simulink subsystem "AnalogInputFiltering"  (R2019b)
settings: Solver=VariableStepAuto  StartTime=0.0  StopTime=10.0  RelTol=1e-3
undefined symbols (not defined in the file): boardTempTemperatureCal_mC, boardTempVoltageCal_mV, motorDriverTempTemperatureCal_mC, motorDriverTempVoltageCal_mV, throttlePos1Max_cnt, throttlePos1Min_cnt, throttlePos2Max_cnt, throttlePos2Min_cnt
libraries: eeGeneralControl x2, Map x2, dspstat3 x2
settings Model: Creator=Nick  LastModifiedBy=Nick

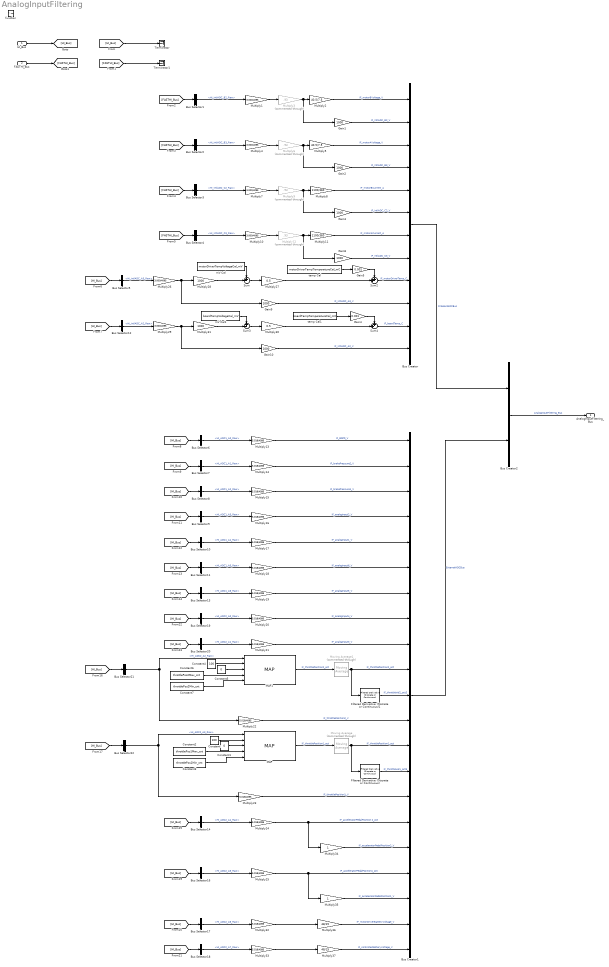
== system AnalogInputFiltering ==
  HI_Bus : Inport
  FASTHI_Bus : Inport  Port=2
  function : TriggerPort  TriggerType=function-call  VariantControl=Variant
  Bus Creator : BusCreator  Inputs=12
  Bus Creator1 : BusCreator  Inputs=21
  Bus Creator2 : BusCreator  Inputs=2
  Bus Selector1 : BusSelector  OutputSignals=HI_intlADC_B2_Raw
  Bus Selector10 : BusSelector  OutputSignals=SPIBus.ADC1Bus.HI_ADC1_A4_Raw
  Bus Selector11 : BusSelector  OutputSignals=SPIBus.ADC1Bus.HI_ADC1_A5_Raw
  Bus Selector12 : BusSelector  OutputSignals=AnalogBus.HI_intlADC_A2_Raw
  Bus Selector13 : BusSelector  OutputSignals=SPIBus.ADC1Bus.HI_ADC1_A6_Raw
  Bus Selector14 : BusSelector  OutputSignals=SPIBus.ADC2Bus.HI_ADC2_A4_Raw
  Bus Selector16 : BusSelector  OutputSignals=SPIBus.ADC2Bus.HI_ADC2_A5_Raw
  Bus Selector17 : BusSelector  OutputSignals=SPIBus.ADC2Bus.HI_ADC2_A6_Raw
  Bus Selector18 : BusSelector  OutputSignals=SPIBus.ADC2Bus.HI_ADC2_A7_Raw
  Bus Selector19 : BusSelector  OutputSignals=SPIBus.ADC2Bus.HI_ADC2_A0_Raw
  Bus Selector2 : BusSelector  OutputSignals=HI_intlADC_B3_Raw
  Bus Selector20 : BusSelector  OutputSignals=SPIBus.ADC2Bus.HI_ADC2_A1_Raw
  Bus Selector21 : BusSelector  OutputSignals=SPIBus.ADC2Bus.HI_ADC2_A2_Raw
  Bus Selector22 : BusSelector  OutputSignals=SPIBus.ADC2Bus.HI_ADC2_A3_Raw
  Bus Selector3 : BusSelector  OutputSignals=HI_intlADC_C2_Raw
  Bus Selector4 : BusSelector  OutputSignals=HI_intlADC_C3_Raw
  Bus Selector5 : BusSelector  OutputSignals=AnalogBus.HI_intlADC_A3_Raw
  Bus Selector6 : BusSelector  OutputSignals=SPIBus.ADC1Bus.HI_ADC1_A0_Raw
  Bus Selector7 : BusSelector  OutputSignals=SPIBus.ADC1Bus.HI_ADC1_A1_Raw
  Bus Selector8 : BusSelector  OutputSignals=SPIBus.ADC1Bus.HI_ADC1_A2_Raw
  Bus Selector9 : BusSelector  OutputSignals=SPIBus.ADC1Bus.HI_ADC1_A3_Raw
  Constant : Constant  Value=100
  Constant1 : Constant  Value=0
  Constant2 : Constant  Value=throttlePos1Max_cnt
  Constant3 : Constant  Value=throttlePos1Min_cnt
  Constant4 : Constant  Value=100
  Constant5 : Constant  Value=0
  Constant6 : Constant  Value=throttlePos2Max_cnt
  Constant7 : Constant  Value=throttlePos2Min_cnt
  Filtered Derivative (Discrete or Continuous) : eeGeneralControl/Filtered Derivative (Discrete or Continuous)  K=1  T=0.01  B=inf  A=-inf  minRatio=10  Ts=-1
      settings: SourceProductName=Simscape Electrical  SourceProductBaseCode=PS
  Filtered Derivative (Discrete or Continuous)1 : eeGeneralControl/Filtered Derivative (Discrete or Continuous)  K=1  T=0.01  B=inf  A=-inf  minRatio=10  Ts=-1
      settings: SourceProductName=Simscape Electrical  SourceProductBaseCode=PS
  Gain{1..3,8..10} (6 alike) : Gain  Gain=1000
  Gain4 : Gain  Gain=0.001
  Gain5 : Gain  Gain=0.001
  MAP : Map/Algroithms/MAP  SystemSampleTime=-1  Latency=0  AutoFrameSizeCalculation=off
  MAP1 : Map/Algroithms/MAP  SystemSampleTime=-1  Latency=0  AutoFrameSizeCalculation=off
  Moving Average : dspstat3/Moving Average  Commented=through  Method=Sliding window  ForgettingFactorPort=off  SpecifyWindowLength=on  WindowLength=10  ForgettingFactor=0.9  SimulateUsing=Code generation
  Moving Average1 : dspstat3/Moving Average  Commented=through  Method=Sliding window  ForgettingFactorPort=off  SpecifyWindowLength=on  WindowLength=10  ForgettingFactor=0.9  SimulateUsing=Code generation
  Multiply{1,4,7,10} (4 alike) : Gain  Gain=3.000/4095
  Multiply11 : Gain  Gain=1100/360
  Multiply{3,6,9,12} (4 alike) : Gain  Commented=through  Gain=.93
  Multiply{13..25,32..33} (15 alike) : Gain  Gain=5.018/4095  OutDataTypeStr=double
  Multiply2 : Gain  Gain=40.5/7.5
  Multiply26 : Gain  Gain=3.000/4095  OutDataTypeStr=double
  Multiply27 : Gain  Gain=0.5
  Multiply28 : Gain  Gain=1000  OutDataTypeStr=double
  Multiply29 : Gain  Gain=3.000/4095  OutDataTypeStr=double
  Multiply30 : Gain  Gain=0.5
  Multiply31 : Gain  Gain=1000  OutDataTypeStr=double
  Multiply34 : Gain  OutDataTypeStr=double
  Multiply35 : Gain  OutDataTypeStr=double
  Multiply36 : Gain  Gain=48/15  OutDataTypeStr=double
  Multiply37 : Gain  Gain=48/15  OutDataTypeStr=double
  Multiply5 : Gain  Gain=40.5/7.5
  Multiply8 : Gain  Gain=1100/360
  Sum : Sum  Inputs=+-|
  Sum2 : Sum  Inputs=++|
  Sum3 : Sum  Inputs=+-|
  Sum4 : Sum  Inputs=++|
  Terminator : Terminator
  Terminator1 : Terminator
  mV Cal : Constant  Value=motorDriverTempVoltageCal_mV
  mV Cal1 : Constant  Value=boardTempVoltageCal_mV
  temp Cal : Constant  Value=motorDriverTempTemperatureCal_mC
  temp Cal1 : Constant  Value=boardTempTemperatureCal_mC
  AnalogInputFiltering_Bus : Outport
  wires:
  Multiply34/1 -> Bus Creator1/17  "IF_acceleratorPedalPosition2_V"
  Multiply35/1 -> Bus Creator1/19  "IF_acceleratorPedalPosition1_V"
  Multiply13/1 -> Bus Creator1/1  "IF_BSPD_V"
  Sum4/1 -> Bus Creator/11  "IF_boardTemp_C"
  Multiply29/1 -> Gain10/1, Multiply31/1
  Multiply30/1 -> Sum4/2
  Gain10/1 -> Bus Creator/12  "IF_intlADC_A2_V"
  Sum3/1 -> Multiply30/1
  mV Cal1/1 -> Sum3/1
  Sum2/1 -> Bus Creator/9  "IF_motorDriverTemp_C"
  temp Cal/1 -> Gain5/1
  Sum/1 -> Multiply27/1
  mV Cal/1 -> Sum/1
  Bus Selector12/1 -> Multiply29/1  "<HI_intlADC_A2_Raw>"
  [HI_Bus] -> Bus Selector12/1
  Bus Selector5/1 -> Multiply26/1  "<HI_intlADC_A3_Raw>"
  [HI_Bus] -> Bus Selector5/1
  Gain9/1 -> Bus Creator/10  "IF_intlADC_A3_V"
  Multiply27/1 -> Sum2/2
  Multiply26/1 -> Gain9/1, Multiply28/1
  Multiply12/1 -> Multiply11/1, Gain8/1
  Multiply11/1 -> Bus Creator/7  "IF_motorACurrent_A"
  Multiply10/1 -> Multiply12/1
  [FASTHI_Bus] -> Bus Selector4/1
  Bus Selector4/1 -> Multiply10/1  "<HI_intlADC_C3_Raw>"
  Gain8/1 -> Bus Creator/8  "IF_intlADC_C3_V"
  Multiply8/1 -> Bus Creator/5  "IF_motorBCurrent_A"
  Gain3/1 -> Bus Creator/6  "IF_intlADC_C2_V"
  Bus Selector3/1 -> Multiply7/1  "<HI_intlADC_C2_Raw>"
  Multiply7/1 -> Multiply9/1
  Multiply9/1 -> Multiply8/1, Gain3/1
  [FASTHI_Bus] -> Bus Selector3/1
  Gain2/1 -> Bus Creator/4  "IF_intlADC_B3_V"
  [FASTHI_Bus] -> Bus Selector2/1
  Bus Selector2/1 -> Multiply4/1  "<HI_intlADC_B3_Raw>"
  Multiply5/1 -> Bus Creator/3  "IF_motorAVoltage_V"
  Multiply4/1 -> Multiply6/1
  Multiply6/1 -> Multiply5/1, Gain2/1
  Multiply3/1 -> Multiply2/1, Gain1/1
  Bus Selector1/1 -> Multiply1/1  "<HI_intlADC_B2_Raw>"
  Multiply1/1 -> Multiply3/1
  Multiply2/1 -> Bus Creator/1  "IF_motorBVoltage_V"
  [FASTHI_Bus] -> Bus Selector1/1
  Gain1/1 -> Bus Creator/2  "IF_intlADC_B2_V"
  FASTHI_Bus/1 -> [FASTHI_Bus]
  [FASTHI_Bus] -> Terminator1/1
  [HI_Bus] -> Terminator/1
  HI_Bus/1 -> [HI_Bus]
  Bus Creator2/1 -> AnalogInputFiltering_Bus/1  "AnalogInputFiltering_Bus"
  Bus Creator/1 -> Bus Creator2/1  "OnboardADCBus"
  Bus Creator1/1 -> Bus Creator2/2  "ExternalADCBus"
  [HI_Bus] -> Bus Selector6/1
  Bus Selector6/1 -> Multiply13/1  "<HI_ADC1_A0_Raw>"
  Bus Selector7/1 -> Multiply14/1  "<HI_ADC1_A1_Raw>"
  [HI_Bus] -> Bus Selector7/1
  Multiply14/1 -> Bus Creator1/2  "IF_brakePressure2_V"
  Bus Selector8/1 -> Multiply15/1  "<HI_ADC1_A2_Raw>"
  Multiply15/1 -> Bus Creator1/3  "IF_brakePressure1_V"
  [HI_Bus] -> Bus Selector8/1
  Bus Selector9/1 -> Multiply16/1  "<HI_ADC1_A3_Raw>"
  Multiply16/1 -> Bus Creator1/4  "IF_analogInput2_V"
  [HI_Bus] -> Bus Selector9/1
  Bus Selector10/1 -> Multiply17/1  "<HI_ADC1_A4_Raw>"
  Multiply17/1 -> Bus Creator1/5  "IF_analogInput1_V"
  [HI_Bus] -> Bus Selector10/1
  Bus Selector11/1 -> Multiply18/1  "<HI_ADC1_A5_Raw>"
  Multiply18/1 -> Bus Creator1/6  "IF_analogInput6_V"
  [HI_Bus] -> Bus Selector11/1
  Bus Selector13/1 -> Multiply19/1  "<HI_ADC1_A6_Raw>"
  Multiply19/1 -> Bus Creator1/7  "IF_analogInput5_V"
  [HI_Bus] -> Bus Selector13/1
  Bus Selector19/1 -> Multiply20/1  "<HI_ADC2_A0_Raw>"
  [HI_Bus] -> Bus Selector21/1
  [HI_Bus] -> Bus Selector17/1
  Multiply32/1 -> Multiply36/1
  Multiply20/1 -> Bus Creator1/8  "IF_analogInput4_V"
  Bus Selector17/1 -> Multiply32/1  "<HI_ADC2_A6_Raw>"
  [HI_Bus] -> Bus Selector20/1
  [HI_Bus] -> Bus Selector19/1
  Multiply21/1 -> Bus Creator1/9  "IF_analogInput3_V"
  Bus Selector20/1 -> Multiply21/1  "<HI_ADC2_A1_Raw>"
  Multiply33/1 -> Multiply37/1
  [HI_Bus] -> Bus Selector16/1
  Bus Selector16/1 -> Multiply25/1  "<HI_ADC2_A5_Raw>"
  Multiply25/1 -> Multiply35/1, Bus Creator1/18  "IF_acceleratorPedalPosition1_pct"
  Bus Selector18/1 -> Multiply33/1  "<HI_ADC2_A7_Raw>"
  Multiply23/1 -> Bus Creator1/15  "IF_throttlePosition1_V"
  Multiply22/1 -> Bus Creator1/12  "IF_throttlePosition2_V"
  [HI_Bus] -> Bus Selector18/1
  Bus Selector22/1 -> Multiply23/1, MAP/1  "<HI_ADC2_A3_Raw>"
  [HI_Bus] -> Bus Selector22/1
  Filtered Derivative (Discrete or Continuous)/1 -> Bus Creator1/14  "IF_throttleVel1_pctS"
  Moving Average/1 -> Filtered Derivative (Discrete or Continuous)/1, Bus Creator1/13  "IF_throttlePosition1_pct"
  MAP/1 -> Moving Average/1  "IF_throttlePosition1_pct"
  Multiply24/1 -> Multiply34/1, Bus Creator1/16  "IF_acceleratorPedalPosition 2_pct"
  [HI_Bus] -> Bus Selector14/1
  Bus Selector14/1 -> Multiply24/1  "<HI_ADC2_A4_Raw>"
  Bus Selector21/1 -> Multiply22/1, MAP1/1  "<HI_ADC2_A2_Raw>"
  Filtered Derivative (Discrete or Continuous)1/1 -> Bus Creator1/11  "IF_throttleVel2_pctS"
  MAP1/1 -> Moving Average1/1  "IF_throttlePosition2_pct"
  Moving Average1/1 -> Filtered Derivative (Discrete or Continuous)1/1, Bus Creator1/10  "IF_throttlePosition2_pct"
  Multiply36/1 -> Bus Creator1/20  "IF_motorDriverBatteryVoltage_V"
  Multiply37/1 -> Bus Creator1/21  "IF_controllerBatteryVoltage_V"
  Multiply28/1 -> Sum/2
  Multiply31/1 -> Sum3/2
  temp Cal1/1 -> Gain4/1
  Gain4/1 -> Sum4/1
  Gain5/1 -> Sum2/1
  Constant2/1 -> MAP/4
  Constant1/1 -> MAP/3
  Constant/1 -> MAP/2
  Constant3/1 -> MAP/5
  Constant6/1 -> MAP1/4
  Constant7/1 -> MAP1/5
  Constant4/1 -> MAP1/2
  Constant5/1 -> MAP1/3
